simulink model "AccumulatorManagementRing"  (R2020a)
settings: Solver=FixedStepDiscrete  StartTime=0.0  StopTime=10.0  FixedStep=ModelSimTime  MaxStep=Ts  RelTol=1e-3
PostLoadFcn:
  | , if any(exist('dsrtsu_mdlpostloadfcn', 'file') ~= 0), dsrtsu_mdlpostloadfcn('Execute', bdroot); end,
undefined symbols (not defined in the file): AMR, ModelSimTime, RING_STATUS
libraries: moving_average x2, discrete_timer x2, commutil2 x1, simulink x1
settings Model: DSRTSU_INTERNAL_RTI_VER=530  DSRTSU_INTERNAL_RTI_TYPE=rti1401  RTICANMMDATA=struct('GeneralSetupData',struct('modelroot','C:\Users\harjo\Git\MACFormulaGit\MicroAutobox\rings\Accumulator_Management_Ring','generalsettings',struct('filesettings',struct('destfolder',struct('Name','RTICANMM_FILES','Check',1),'buildfolder',struct('Name','.','Check',1),'AbsDestfolder',struct('Name','C:\Users\harjo\Git\MACFormulaGit\MicroAutobox\rings\Accumulator_Management_Ring\RTICANMM_FILES'),'AbsBuildfolder',struct('Name','C:\Users\harjo\Git\MACFormulaGit\MicroAutobox\rings\Accumulator_Management_Ring'))),'options',struct('addpaths',1,'rmpaths',1,'addtrcexclusion',logical(1),'cannavigator',struct('checkmonitoring',0),'show_usrtrc',0,'use_usrtrc',0),'advanced',struct('options',ones(1,100)),'MPSetup',{{}},'RTI',struct('Type','GRT','Ver','','Date',''),'modelname','AccumulatorManagementRing','block','AccumulatorManagementRing'))  DSRTSU_INTERNAL_RTIFPGA=120  Creator=Harjot  LastModifiedBy=harjo
settings DataIOCC: SaveOutput=off  SaveTime=off  ReturnWorkspaceOutputs=off
settings OptimizationCC: EfficientMapNaN2IntZero=off
settings DebuggingCC: ArithmeticOperatorsInVariantConditions=warning
settings HardwareCC: ProdBitPerPointer=32  ProdBitPerSizeT=32  ProdBitPerPtrDiffT=32  ProdLargestAtomicInteger=Integer  ProdEndianess=BigEndian  ProdWordSize=32  ProdHWDeviceType=Custom Processor->Custom  TargetBitPerPointer=64  TargetLargestAtomicInteger=Integer  TargetLongLongMode=on  TargetIntDivRoundTo=Zero  TargetEndianess=BigEndian  TargetHWDeviceType=Custom Processor->Custom
settings SFSimCC: SimUseLocalCustomCode=off  MATLABDynamicMemAlloc=off  CustomCodeUndefinedFunction=UseInterfaceOnly
settings RTWCC: Description=dSPACE DS1401 Hardware Platform  SystemTargetFile=rti1401.tlc  MakeCommand=make_rti  TemplateMakefile=rti1401.tmf
settings CodeAppCC: MaxIdLength=128
settings STFCustomTargetCC: UtilityFuncGeneration=Shared location  ParMdlRefBuildCompliant=on  SystemTargetFile=rti1401.tlc
settings GRTTargetCC: TargetLangStandard=C89/C90 (ANSI)  UtilityFuncGeneration=Shared location  CompOptLevelCompliant=off  ConcurrentExecutionCompliant=off  CombineOutputUpdateFcns=off  MatFileLogging=off  CPPClassGenCompliant=off  UseToolchainInfoCompliant=off

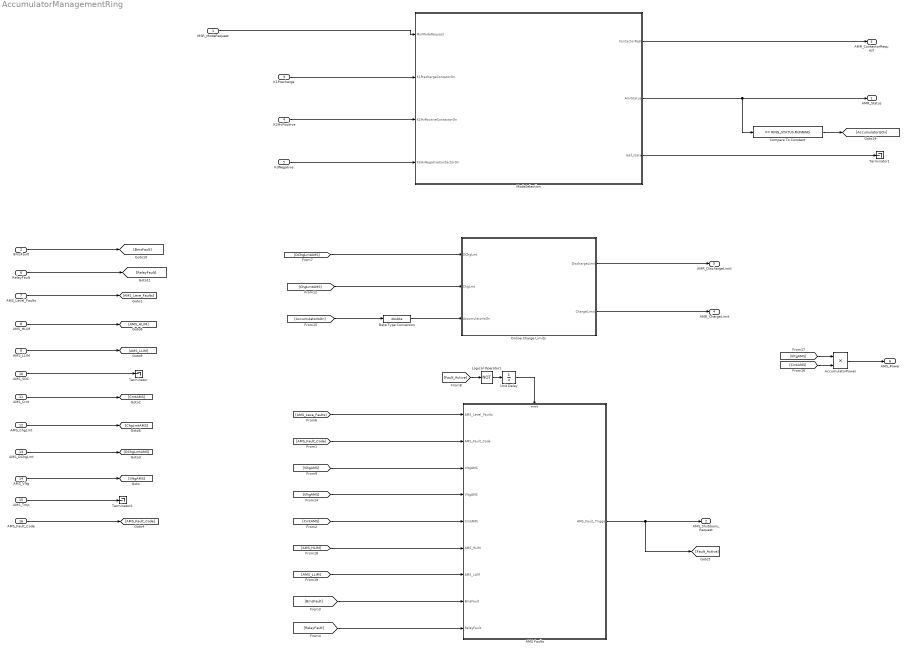
== system AccumulatorManagementRing ==
  MSR_ModeRequest : Inport
  BmsFault : Inport  Port=2
  K1Precharge : Inport  Port=3
  K2HvPositive : Inport  Port=4
  K3Negative : Inport  Port=5
  RelayFault : Inport  Port=6
  AMS_Level_Faults : Inport  Port=7  OutDataTypeStr=uint8
  AMS_HLIM : Inport  Port=8
  AMS_LLIM : Inport  Port=9
  AMS_SOC : Inport  Port=10
  AMS_Crnt : Inport  Port=11
  AMS_ChgLmt : Inport  Port=12  OutDataTypeStr=double
  AMS_DChgLmt : Inport  Port=13  OutDataTypeStr=double
  AMS_Vltg : Inport  Port=14
  AMS_Tmp : Inport  Port=15
  AMS_Fault_Code : Inport  Port=16  OutDataTypeStr=uint8
  " ModeSelection" : Stateflow chart  TreatAsAtomicUnit=on
  AMS Faults : Subsystem
  AccumulatorPower : Product
  Compare To Constant : simulink/Logic and Bit Operations/Compare To Constant  relop===  const=RING_STATUS.RUNNING  OutDataTypeStr=boolean
  Data Type Conversion : DataTypeConversion  OutDataTypeStr=double
  Logical Operator1 : Logic  Operator=NOT  AllPortsSameDT=off  OutDataTypeStr=boolean
  Online Charge Limits : Subsystem
  Terminator : Terminator
  Terminator1 : Terminator
  Terminator2 : Terminator
  Unit Delay : UnitDelay  SampleTime=-1  HasFrameUpgradeWarning=on
  AMR_Status : Outport  VectorParamsAs1DForOutWhenUnconnected=off
  AMS_Shutdown_Request : Outport  Port=2  VectorParamsAs1DForOutWhenUnconnected=off
  AMR_ContactorRequest : Outport  Port=3  VectorParamsAs1DForOutWhenUnconnected=off
  AMR_ChargeLimit : Outport  Port=4  VectorParamsAs1DForOutWhenUnconnected=off
  AMR_DischargeLimit : Outport  Port=5  VectorParamsAs1DForOutWhenUnconnected=off
  AMS_Power : Outport  Port=6  VectorParamsAs1DForOutWhenUnconnected=off
  wires:
  [CrntAMS] -> AccumulatorPower/2
  [VltgAMS] -> AccumulatorPower/1
  MSR_ModeRequest/1 -> " ModeSelection"/1(MsrModeRequest)
  [AccumulatorIsOn] -> Data Type Conversion/1
  AMS_SOC/1 -> Terminator/1
  AMS_ChgLmt/1 -> [ChgLmtAMS]
  AMS_Crnt/1 -> [CrntAMS]
  AMS_DChgLmt/1 -> [DChgLmtAMS]
  Online Charge Limits/2(ChargeLimit) -> AMR_ChargeLimit/1
  AMS_LLIM/1 -> [AMS_LLIM]
  AMS_Vltg/1 -> [VltgAMS]
  Online Charge Limits/1(DischargeLimit) -> AMR_DischargeLimit/1
  [ChgLmtAMS] -> Online Charge Limits/2(ChgLmt)
  AMS_Tmp/1 -> Terminator2/1
  " ModeSelection"/3(leaf_state) -> Terminator1/1
  [DChgLmtAMS] -> Online Charge Limits/1(DChgLmt)
  AccumulatorPower/1 -> AMS_Power/1
  AMS_HLIM/1 -> [AMS_HLIM]
  " ModeSelection"/1(ContactorRqst) -> AMR_ContactorRequest/1
  " ModeSelection"/2(AmrStatus) -> Compare To Constant/1, AMR_Status/1
  K1Precharge/1 -> " ModeSelection"/2(K1PrechargeContatorOn)
  K2HvPositive/1 -> " ModeSelection"/3(K2HvPositiveContactorOn)
  K3Negative/1 -> " ModeSelection"/4(K3HvNegativeContactorOn)
  Compare To Constant/1 -> [AccumulatorIsOn]
  AMS_Level_Faults/1 -> [AMS_Leve_Faults]
  AMS_Fault_Code/1 -> [AMS_Fault_Code]
  [AMS_Fault_Code] -> AMS Faults/2(AMS_Fault_Code)
  [VltgAMS] -> AMS Faults/3("VltgAMS ")
  Unit Delay/1 -> AMS Faults/Enable
  AMS Faults/1("AMS_Fault_Trigger ") -> AMS_Shutdown_Request/1, [Fault_Active]
  [Fault_Active] -> Logical Operator1/1
  [AMS_HLIM] -> AMS Faults/6(AMS_HLIM)
  [VltgAMS] -> AMS Faults/4(VltgAMS)
  [CrntAMS] -> AMS Faults/5(CrntAMS)
  Logical Operator1/1 -> Unit Delay/1
  [AMS_Leve_Faults] -> AMS Faults/1(AMS_Level_Faults)
  [AMS_LLIM] -> AMS Faults/7(AMS_LLIM)
  BmsFault/1 -> [BmsFault]
  RelayFault/1 -> [RelayFault]
  [BmsFault] -> AMS Faults/8(BmsFault)
  [RelayFault] -> AMS Faults/9(RelayFault)
  Data Type Conversion/1 -> Online Charge Limits/3(AccumulatorIsOn)

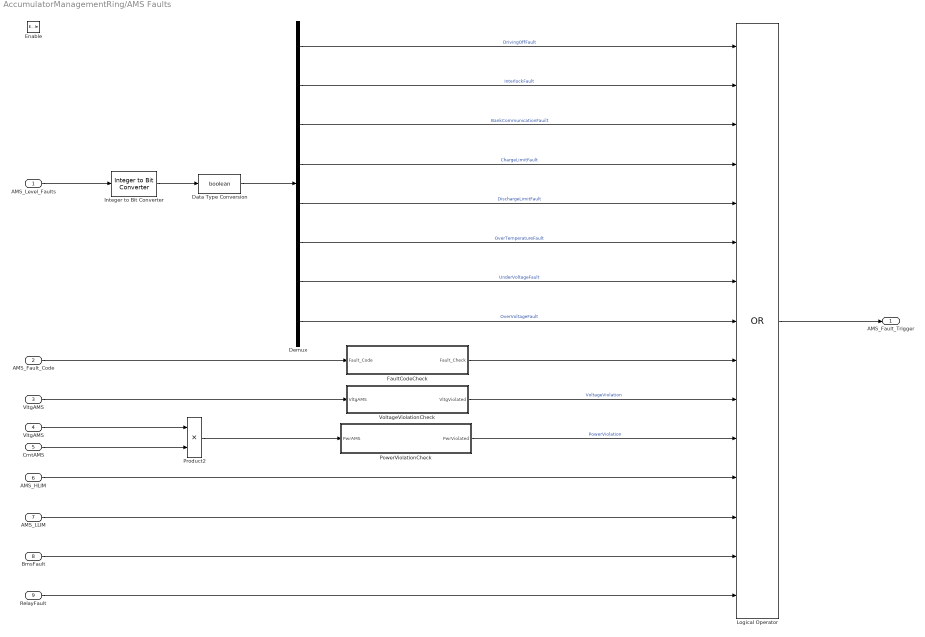
== system AccumulatorManagementRing/AMS Faults ==
  AMS_Level_Faults : Inport
  AMS_Fault_Code : Inport  Port=2
  "VltgAMS " : Inport  Port=3
  VltgAMS : Inport  Port=4
  CrntAMS : Inport  Port=5
  AMS_HLIM : Inport  Port=6
  AMS_LLIM : Inport  Port=7
  BmsFault : Inport  Port=8
  RelayFault : Inport  Port=9
  Enable : EnablePort
  Data Type Conversion : DataTypeConversion  OutDataTypeStr=boolean
  Demux : Demux  Outputs=8
  FaultCodeCheck : Subsystem
  Integer to Bit Converter : commutil2/Integer to Bit Converter  nbits=8  signedInputValues=Unsigned  bitOrder=LSB first  outDtype=Inherit via internal rule
  Logical Operator : Logic  Operator=OR  Inputs=15  AllPortsSameDT=off  OutDataTypeStr=boolean
  "PowerViolationCheck " : Subsystem
  Product2 : Product
  VoltageViolationCheck : Subsystem
  "AMS_Fault_Trigger " : Outport  VectorParamsAs1DForOutWhenUnconnected=off
  wires:
  Integer to Bit Converter/1 -> Data Type Conversion/1
  AMS_Level_Faults/1 -> Integer to Bit Converter/1
  Data Type Conversion/1 -> Demux/1
  AMS_Fault_Code/1 -> FaultCodeCheck/1(Fault_Code)
  Product2/1 -> "PowerViolationCheck "/1(PwrAMS)
  VltgAMS/1 -> Product2/1
  "VltgAMS "/1 -> VoltageViolationCheck/1(VltgAMS)
  CrntAMS/1 -> Product2/2
  Demux/1 -> Logical Operator/1  "DrivingOffFault"
  Demux/2 -> Logical Operator/2  "InterlockFault"
  Demux/3 -> Logical Operator/3  "BankCommunicationFauilt"
  Demux/4 -> Logical Operator/4  "ChargeLimitFault"
  Demux/5 -> Logical Operator/5  "DischargeLimitFault"
  Demux/6 -> Logical Operator/6  "OverTemperatureFault"
  Demux/7 -> Logical Operator/7  "UnderVoltageFault"
  Demux/8 -> Logical Operator/8  "OverVoltageFault"
  FaultCodeCheck/1(Fault_Check) -> Logical Operator/9
  VoltageViolationCheck/1(VltgViolated) -> Logical Operator/10  "VoltageViolation"
  "PowerViolationCheck "/1(PwrViolated) -> Logical Operator/11  "PowerViolation"
  Logical Operator/1 -> "AMS_Fault_Trigger "/1
  AMS_HLIM/1 -> Logical Operator/12
  AMS_LLIM/1 -> Logical Operator/13
  BmsFault/1 -> Logical Operator/14
  RelayFault/1 -> Logical Operator/15

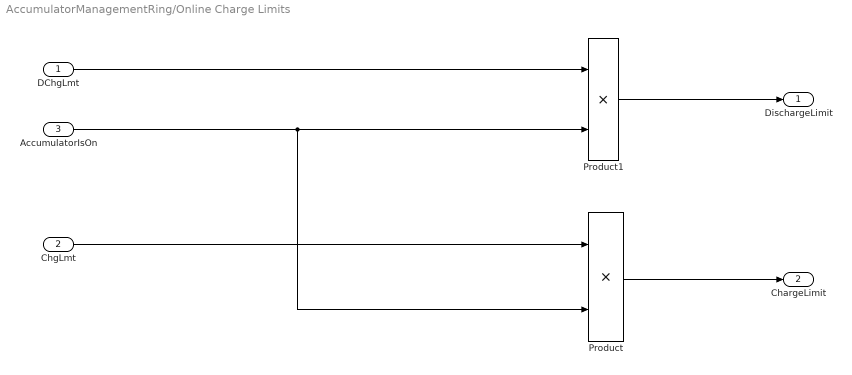
== system AccumulatorManagementRing/Online Charge Limits ==
  DChgLmt : Inport
  ChgLmt : Inport  Port=2
  AccumulatorIsOn : Inport  Port=3
  Product : Product
  Product1 : Product
  DischargeLimit : Outport  VectorParamsAs1DForOutWhenUnconnected=off
  ChargeLimit : Outport  Port=2  VectorParamsAs1DForOutWhenUnconnected=off
  wires:
  AccumulatorIsOn/1 -> Product/2, Product1/2
  ChgLmt/1 -> Product/1
  Product/1 -> ChargeLimit/1
  DChgLmt/1 -> Product1/1
  Product1/1 -> DischargeLimit/1

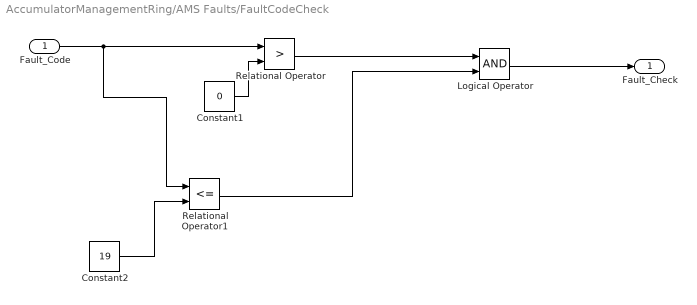
== system AccumulatorManagementRing/AMS Faults/FaultCodeCheck ==
  Fault_Code : Inport
  Constant1 : Constant  Value=0
  Constant2 : Constant  Value=19
  Logical Operator : Logic  AllPortsSameDT=off  OutDataTypeStr=boolean
  Relational Operator : RelationalOperator  Operator=>  OutDataTypeStr=boolean  RndMeth=Simplest
  Relational Operator1 : RelationalOperator  Operator=<=  OutDataTypeStr=boolean  RndMeth=Simplest
  Fault_Check : Outport  VectorParamsAs1DForOutWhenUnconnected=off
  wires:
  Fault_Code/1 -> Relational Operator1/1, Relational Operator/1
  Constant1/1 -> Relational Operator/2
  Constant2/1 -> Relational Operator1/2
  Relational Operator1/1 -> Logical Operator/2
  Relational Operator/1 -> Logical Operator/1
  Logical Operator/1 -> Fault_Check/1

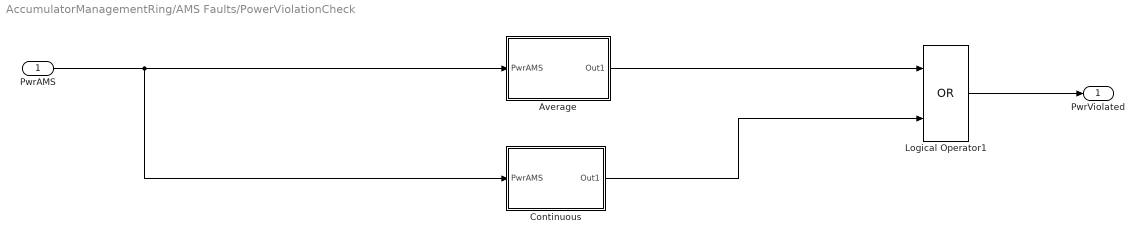
== system AccumulatorManagementRing/AMS Faults/PowerViolationCheck  ==
  PwrAMS : Inport
  Average : Subsystem
  Continuous : Subsystem
  Logical Operator1 : Logic  Operator=OR  AllPortsSameDT=off  OutDataTypeStr=boolean
  PwrViolated : Outport  VectorParamsAs1DForOutWhenUnconnected=off
  wires:
  Logical Operator1/1 -> PwrViolated/1
  PwrAMS/1 -> Continuous/1(PwrAMS), Average/1(PwrAMS)
  Average/1(Out1) -> Logical Operator1/1
  Continuous/1(Out1) -> Logical Operator1/2

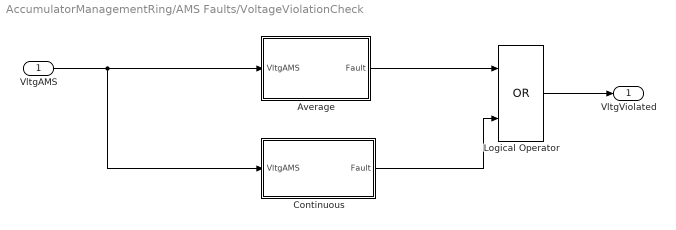
== system AccumulatorManagementRing/AMS Faults/VoltageViolationCheck ==
  VltgAMS : Inport
  Average : Subsystem
  Continuous : Subsystem
  Logical Operator : Logic  Operator=OR  AllPortsSameDT=off  OutDataTypeStr=boolean
  VltgViolated : Outport  VectorParamsAs1DForOutWhenUnconnected=off
  wires:
  Logical Operator/1 -> VltgViolated/1
  Average/1(Fault) -> Logical Operator/1
  Continuous/1(Fault) -> Logical Operator/2
  VltgAMS/1 -> Continuous/1(VltgAMS), Average/1(VltgAMS)

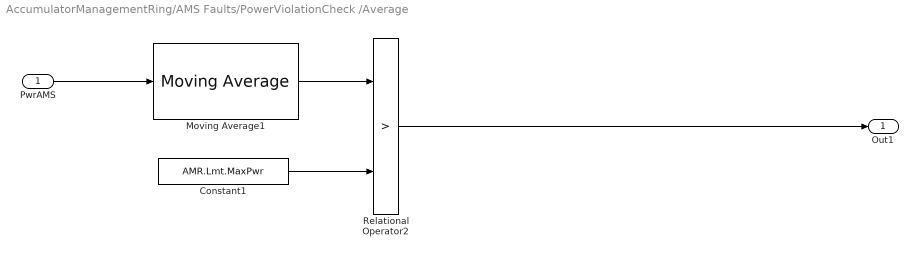
== system AccumulatorManagementRing/AMS Faults/PowerViolationCheck /Average ==
  PwrAMS : Inport
  Constant1 : Constant  Value=AMR.Lmt.MaxPwr
  Moving Average1 : moving_average/Moving Average  SampleTime=ModelSimTime  WindowSize=AMR.Lmt.Tavg
  Relational Operator2 : RelationalOperator  Operator=>  OutDataTypeStr=boolean  RndMeth=Nearest
  Out1 : Outport  VectorParamsAs1DForOutWhenUnconnected=off
  wires:
  Relational Operator2/1 -> Out1/1
  Constant1/1 -> Relational Operator2/2
  Moving Average1/1 -> Relational Operator2/1
  PwrAMS/1 -> Moving Average1/1

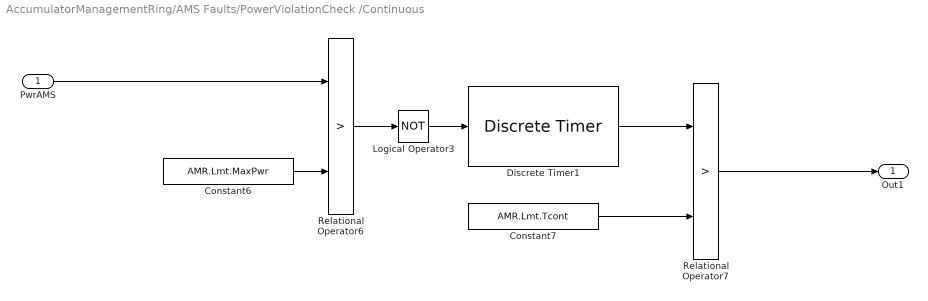
== system AccumulatorManagementRing/AMS Faults/PowerViolationCheck /Continuous ==
  PwrAMS : Inport
  Constant6 : Constant  Value=AMR.Lmt.MaxPwr
  Constant7 : Constant  Value=AMR.Lmt.Tcont
  Discrete Timer1 : discrete_timer/Discrete Timer
  Logical Operator3 : Logic  Operator=NOT  AllPortsSameDT=off  OutDataTypeStr=boolean
  Relational Operator6 : RelationalOperator  Operator=>  OutDataTypeStr=boolean  RndMeth=Nearest
  Relational Operator7 : RelationalOperator  Operator=>  OutDataTypeStr=boolean  RndMeth=Nearest
  Out1 : Outport  VectorParamsAs1DForOutWhenUnconnected=off
  wires:
  Logical Operator3/1 -> Discrete Timer1/1
  Relational Operator7/1 -> Out1/1
  Relational Operator6/1 -> Logical Operator3/1
  Constant6/1 -> Relational Operator6/2
  Discrete Timer1/1 -> Relational Operator7/1
  Constant7/1 -> Relational Operator7/2
  PwrAMS/1 -> Relational Operator6/1

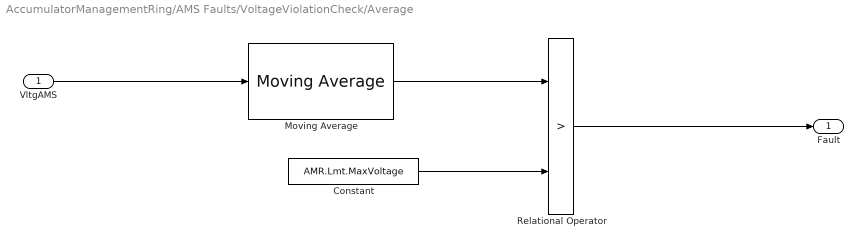
== system AccumulatorManagementRing/AMS Faults/VoltageViolationCheck/Average ==
  VltgAMS : Inport
  Constant : Constant  Value=AMR.Lmt.MaxVoltage
  Moving Average : moving_average/Moving Average  SampleTime=ModelSimTime  WindowSize=AMR.Lmt.Tavg
  Relational Operator : RelationalOperator  Operator=>  OutDataTypeStr=boolean  RndMeth=Nearest
  Fault : Outport  VectorParamsAs1DForOutWhenUnconnected=off
  wires:
  Moving Average/1 -> Relational Operator/1
  VltgAMS/1 -> Moving Average/1
  Constant/1 -> Relational Operator/2
  Relational Operator/1 -> Fault/1

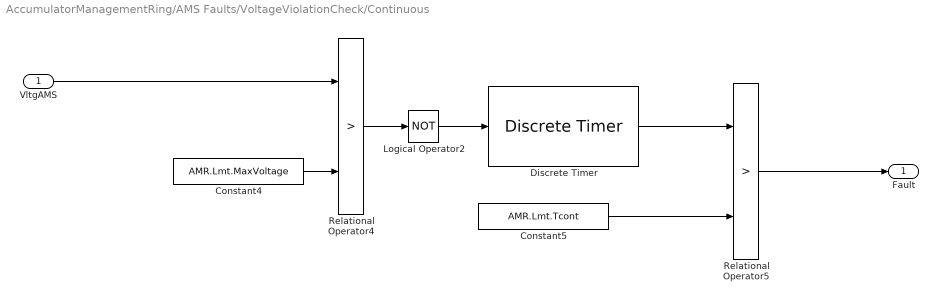
== system AccumulatorManagementRing/AMS Faults/VoltageViolationCheck/Continuous ==
  VltgAMS : Inport
  Constant4 : Constant  Value=AMR.Lmt.MaxVoltage
  Constant5 : Constant  Value=AMR.Lmt.Tcont
  Discrete Timer : discrete_timer/Discrete Timer
  Logical Operator2 : Logic  Operator=NOT  AllPortsSameDT=off  OutDataTypeStr=boolean
  Relational Operator4 : RelationalOperator  Operator=>  OutDataTypeStr=boolean  RndMeth=Nearest
  Relational Operator5 : RelationalOperator  Operator=>  OutDataTypeStr=boolean  RndMeth=Nearest
  Fault : Outport  VectorParamsAs1DForOutWhenUnconnected=off
  wires:
  Logical Operator2/1 -> Discrete Timer/1
  Relational Operator4/1 -> Logical Operator2/1
  Relational Operator5/1 -> Fault/1
  Constant5/1 -> Relational Operator5/2
  Discrete Timer/1 -> Relational Operator5/1
  Constant4/1 -> Relational Operator4/2
  VltgAMS/1 -> Relational Operator4/1

== stateflow chart AccumulatorManagementRing/ ModeSelection ==
  state Off
    entry:
    ContactorRqst = 0;
    AmrStatus = RING_STATUS.OFF;
  state OPERATIONAL
    state Startup
      state RqstPrechg
        entry:
        AmrStatus = RING_STATUS.STARTUP_IN_PROGRESS_HV;
        ContactorRqst = 1;
      state HVPrechg
        entry:
      state HVComplete
        entry:
        AmrStatus = RING_STATUS.STARTUP_COMPLETE_HV;
      (default) -> RqstPrechg
      RqstPrechg -> HVPrechg : [K1PrechargeContatorOn &&...
          | ~K2HvPositiveContactorOn &&...
          | K3HvNegativeContactorOn]
      HVPrechg -> HVComplete : [~K1PrechargeContatorOn &&...
          | K2HvPositiveContactorOn &&...
          | K3HvNegativeContactorOn]
    state Running
      entry:
      AmrStatus = RING_STATUS.RUNNING;
      % No checks are implemented to keep the system as simple as possible
    (default) -> Startup
    Startup -> Running : [MsrModeRequest == MSR_REQUEST.RUNNING && AmrStatus == RING_STATUS.STARTUP_COMPLETE_HV]
  state Shutdown
    en:
    state ShutdownInProgress
      entry:
      AmrStatus = RING_STATUS.SHUTDOWN_IN_PROGRESS_HV;
      ContactorRqst = 0;
    state ShutdownComplete
      entry:
      AmrStatus = RING_STATUS.SHUTDOWN_COMPLETE_HV;
    (default) -> ShutdownInProgress
    ShutdownInProgress -> ShutdownComplete : [~K1PrechargeContatorOn &&...
        | ~K2HvPositiveContactorOn &&...
        | ~K3HvNegativeContactorOn]
  (default) -> Off
  Off -> OPERATIONAL : [MsrModeRequest == MSR_REQUEST.STARTUP_HV]
  OPERATIONAL -> Shutdown : [MsrModeRequest == MSR_REQUEST.SHUTDOWN_HV]
  data: MsrModeRequest input Enum: MSR_REQUEST; ContactorRqst output; K1PrechargeContatorOn input boolean; AmrStatus output Enum: RING_STATUS; leaf_state output Enum: AMR_leaf_states; K2HvPositiveContactorOn input boolean; K3HvNegativeContactorOn input boolean
